simulink model "Lab2_Q19"  (R2023b)
settings: Solver=VariableStepAuto  StartTime=0.0  StopTime=10.0  RelTol=1e-3
libraries: commanabbnd3 x3, dspsrcs4 x2
settings Model: Creator=lijingxuan  LastModifiedBy=lijingxuan

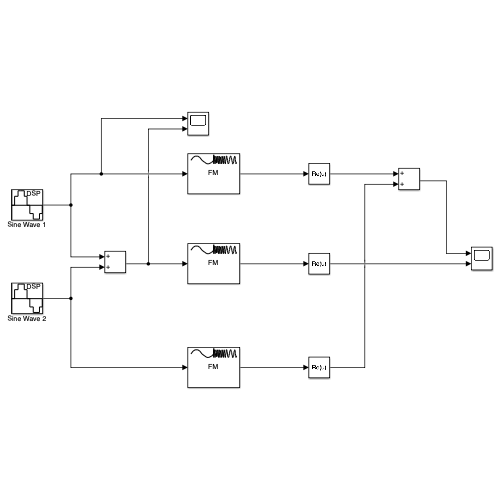
[thumbnail: Simulink's stored preview of the top-level diagram]
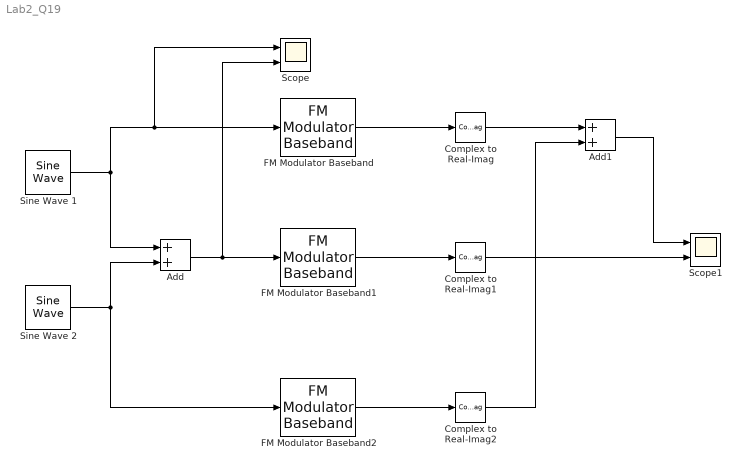
== system Lab2_Q19 ==
  Add : Sum
  Add1 : Sum
  Complex to Real-Imag : ComplexToRealImag  Output=Real
  Complex to Real-Imag1 : ComplexToRealImag  Output=Real
  Complex to Real-Imag2 : ComplexToRealImag  Output=Real
  FM Modulator Baseband : commanabbnd3/FM Modulator Baseband  FrequencyDeviation=50  SimulateUsing=Interpreted execution
  FM Modulator Baseband1 : commanabbnd3/FM Modulator Baseband  FrequencyDeviation=50  SimulateUsing=Interpreted execution
  FM Modulator Baseband2 : commanabbnd3/FM Modulator Baseband  FrequencyDeviation=50  SimulateUsing=Interpreted execution
  Scope : Scope  NumInputPorts=2
  Scope1 : Scope  NumInputPorts=2
  Sine Wave 1 : dspsrcs4/Sine Wave  Amplitude=1  Frequency=4  Phase=0  SampleMode=Discrete  OutComplex=Real  CompMethod=Trigonometric fcn  TableSize=Speed  SampleTime=1/1000  SamplesPerFrame=500  ResetState=Restart at time zero  OutputFrames=off  dataType=double  wordLen=16  udDataType=sfix(16)  fracBitsMode=Best precision  numFracBits=15  OutDataTypeStr=double  LastOutDataTypeStr=double
  Sine Wave 2 : dspsrcs4/Sine Wave  Amplitude=1  Frequency=8  Phase=pi/4  SampleMode=Discrete  OutComplex=Real  CompMethod=Trigonometric fcn  TableSize=Speed  SampleTime=1/1000  SamplesPerFrame=500  ResetState=Restart at time zero  OutputFrames=off  dataType=double  wordLen=16  udDataType=sfix(16)  fracBitsMode=Best precision  numFracBits=15  OutDataTypeStr=double  LastOutDataTypeStr=double
  wires:
  Add1/1 -> Scope1/1
  Complex to Real-Imag1/1 -> Scope1/2
  Complex to Real-Imag2/1 -> Add1/2
  Complex to Real-Imag/1 -> Add1/1
  FM Modulator Baseband1/1 -> Complex to Real-Imag1/1
  FM Modulator Baseband2/1 -> Complex to Real-Imag2/1
  FM Modulator Baseband/1 -> Complex to Real-Imag/1
  Sine Wave 1/1 -> Scope/1, FM Modulator Baseband/1, Add/1
  Sine Wave 2/1 -> FM Modulator Baseband2/1, Add/2
  Add/1 -> Scope/2, FM Modulator Baseband1/1
